simulink model "sf_resolve_signal_object"  (Simulink 7.6)
settings: Solver=FixedStepDiscrete  StartTime=0.0  StopTime=5  FixedStep=1  RelTol=1e-3
PostLoadFcn:
  | load sf_resolve_signal_object_data;
settings Model: Creator=The MathWorks Inc.  ExtModeAutoUpdateStatusClock=off
settings OptimizationCC: InitFltsAndDblsToZero=on  EfficientMapNaN2IntZero=off
settings DebuggingCC: SolverPrmCheckMsg=none  StrictBusMsg=Warning
settings SFSimCC: SimParseCustomCode=off
settings RTWCC: GenerateReport=on  LaunchReport=on

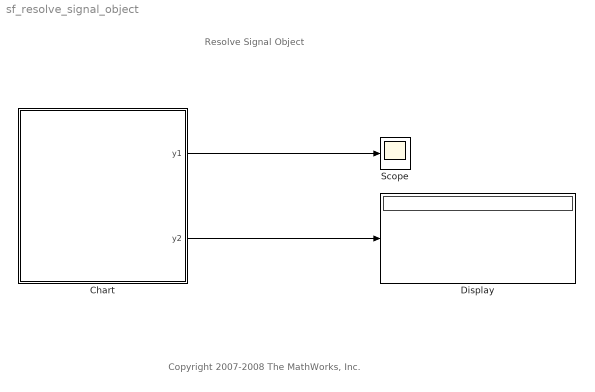
== system sf_resolve_signal_object ==
  note: Resolve Signal Object
  note: Copyright 2007-2008 The MathWorks, Inc.
  Chart : Stateflow chart  TreatAsAtomicUnit=on
  Display : Display
  Scope : Scope
      settings: YMin=15  YMax=17
  wires:
  Chart/1(y1) -> Scope/1
  Chart/2(y2) -> Display/1

== stateflow chart Chart ==
  state S
    en: y1 = 2 * (local + 10);
    du: y2 = 5;
  (default) -> S
  data: local local double; y1 output double; y2 output double
